simulink model "LAB1_5_perSimo"  (R2024b)
settings: Solver=VariableStepAuto  StartTime=0.0  StopTime=5  RelTol=1e-3
values from neighbouring files (symbols this model uses):
  A_ex = [A_p zeros(3,2) ... (first row only)    [LAB1_Corretto.m]
  B_e = [0;B]    [LAB1_Corretto.m]    (also in LAB1_GIOI.m)
  Beq = B_eq_est    [LAB1_Corretto.m]    (also in LAB1_GIOI.m)
  C_ex = [0 0 0 C]    [LAB1_Corretto.m]
  Jeq = J_eq_est    [LAB1_Corretto.m]    (also in LAB1_GIOI.m)
  L_ex = K_ex'    [LAB1_Corretto.m]
  Tausf = tau_sf_est    [LAB1_Corretto.m]    (also in LAB1_GIOI.m)
  w0 = 2*pi/Tr    (= 12.5663706144)    [LAB1_Corretto.m]    (also in LAB1_GIOI.m)
undefined symbols (not defined in the file or in its folder): daq, drv, gbox, mot, pulse2deg, rads2rpm, Req
settings Model: Creator=Gioele  LastModifiedBy=Gioele
settings ConfigComp: CovBoundaryAbsTol=1.0e-5

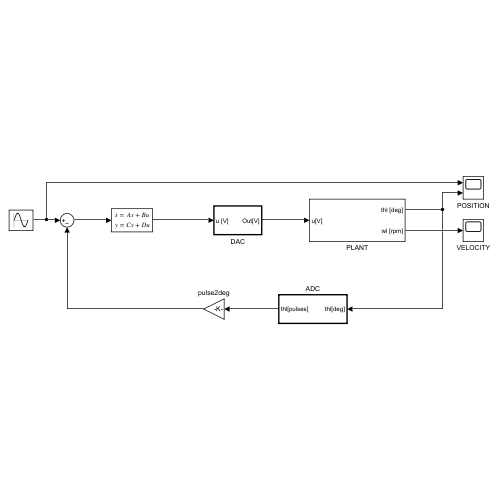
[thumbnail: Simulink's stored preview of the top-level diagram]
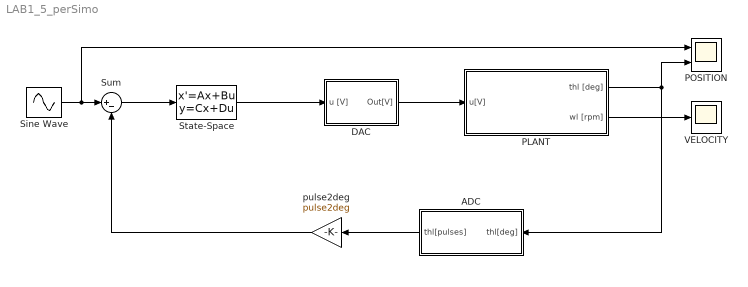
== system LAB1_5_perSimo ==
  ADC : Subsystem  TreatAsAtomicUnit=on
  DAC : Subsystem  TreatAsAtomicUnit=on
  PLANT : Subsystem
  POSITION : Scope  NumInputPorts=2
  Sine Wave : Sin  Amplitude=30  Frequency=w0  SampleTime=0
  State-Space : StateSpace  A=A_ex-L_ex*C_ex  B=[B_e, L_ex]  C=eye(5)  D=0  InitialCondition=0
  Sum : Sum  Inputs=|+-
  VELOCITY : Scope
  pulse2deg : Gain  Gain=pulse2deg
  wires:
  pulse2deg/1 -> Sum/2
  ADC/1(thl[pulses]) -> pulse2deg/1
  Sum/1 -> State-Space/1
  PLANT/1(thl [deg]) -> ADC/1(thl[deg]), POSITION/2
  PLANT/2(wl [rpm]) -> VELOCITY/1
  DAC/1(Out[V]) -> PLANT/1(u[V])
  Sine Wave/1 -> POSITION/1, Sum/1
  State-Space/1 -> DAC/1(u [V])

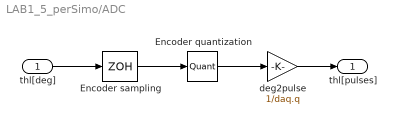
== system LAB1_5_perSimo/ADC ==
  thl[deg] : Inport
  Encoder quantization : Quantizer  QuantizationInterval=daq.q
  Encoder sampling : ZeroOrderHold  SampleTime=daq.dac.Ts
  deg2pulse : Gain  Gain=1/daq.q
  thl[pulses] : Outport
  wires:
  Encoder quantization/1 -> deg2pulse/1
  thl[deg]/1 -> Encoder sampling/1
  Encoder sampling/1 -> Encoder quantization/1
  deg2pulse/1 -> thl[pulses]/1

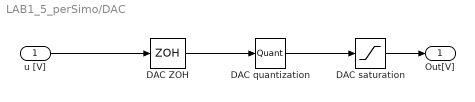
== system LAB1_5_perSimo/DAC ==
  u [V] : Inport
  "DAC ZOH " : ZeroOrderHold  SampleTime=daq.dac.Ts
  DAC quantization : Quantizer  QuantizationInterval=daq.dac.q
  DAC saturation : Saturate  UpperLimit=daq.dac.fs  LowerLimit=-daq.dac.fs
  Out[V] : Outport
  wires:
  DAC quantization/1 -> DAC saturation/1
  u [V]/1 -> "DAC ZOH "/1
  "DAC ZOH "/1 -> DAC quantization/1
  DAC saturation/1 -> Out[V]/1

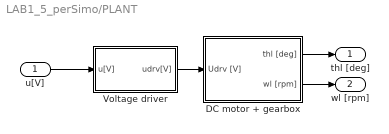
== system LAB1_5_perSimo/PLANT ==
  u[V] : Inport
  DC motor + gearbox : Subsystem
  Voltage driver : Subsystem  TreatAsAtomicUnit=on
  thl [deg] : Outport
  wl [rpm] : Outport  Port=2
  wires:
  Voltage driver/1(udrv[V]) -> DC motor + gearbox/1(Udrv [V])
  DC motor + gearbox/2(wl [rpm]) -> wl [rpm]/1
  DC motor + gearbox/1(thl [deg]) -> thl [deg]/1
  u[V]/1 -> Voltage driver/1(u[V])

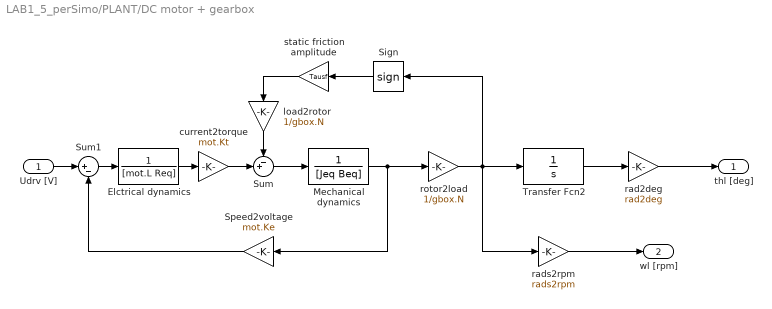
== system LAB1_5_perSimo/PLANT/DC motor + gearbox ==
  Udrv [V] : Inport
  Elctrical dynamics : TransferFcn  Denominator=[mot.L Req]
  Mechanical dynamics : TransferFcn  Denominator=[Jeq Beq]
  Sign : Signum  ZeroCross=off
  Speed2voltage : Gain  Gain=mot.Ke
  Sum : Sum  Inputs=-+|
  Sum1 : Sum  Inputs=|+-
  Transfer Fcn2 : TransferFcn  Denominator=[1 0]
  current2torque : Gain  Gain=mot.Kt
  load2rotor : Gain  Gain=1/gbox.N
  rad2deg : Gain  Gain=rad2deg
  rads2rpm : Gain  Gain=rads2rpm
  rotor2load : Gain  Gain=1/gbox.N
  static friction amplitude : Gain  Gain=Tausf
  thl [deg] : Outport
  wl [rpm] : Outport  Port=2
  wires:
  rotor2load/1 -> Sign/1, rads2rpm/1, Transfer Fcn2/1
  Sign/1 -> static friction amplitude/1
  rads2rpm/1 -> wl [rpm]/1
  Sum/1 -> Mechanical dynamics/1
  Udrv [V]/1 -> Sum1/1
  static friction amplitude/1 -> load2rotor/1
  load2rotor/1 -> Sum/1
  Transfer Fcn2/1 -> rad2deg/1
  current2torque/1 -> Sum/2
  Speed2voltage/1 -> Sum1/2
  Mechanical dynamics/1 -> Speed2voltage/1, rotor2load/1
  Elctrical dynamics/1 -> current2torque/1
  Sum1/1 -> Elctrical dynamics/1
  rad2deg/1 -> thl [deg]/1

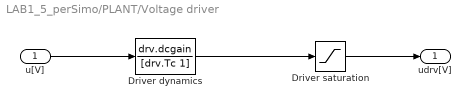
== system LAB1_5_perSimo/PLANT/Voltage driver ==
  u[V] : Inport  OutMax=[5]
  Driver dynamics : TransferFcn  Numerator=drv.dcgain  Denominator=[drv.Tc 1]
  Driver saturation : Saturate  UpperLimit=drv.outmax  LowerLimit=-drv.outmax
  udrv[V] : Outport
  wires:
  Driver dynamics/1 -> Driver saturation/1
  u[V]/1 -> Driver dynamics/1
  Driver saturation/1 -> udrv[V]/1
